simulink model "orbit_propogator_simulink"  (R2023b)
settings: Solver=FixedStepAuto  StartTime=0  StopTime=5929*3  FixedStep=50  RelTol=1e-3
settings Model: Creator=annahylbert  LastModifiedBy=annahylbert

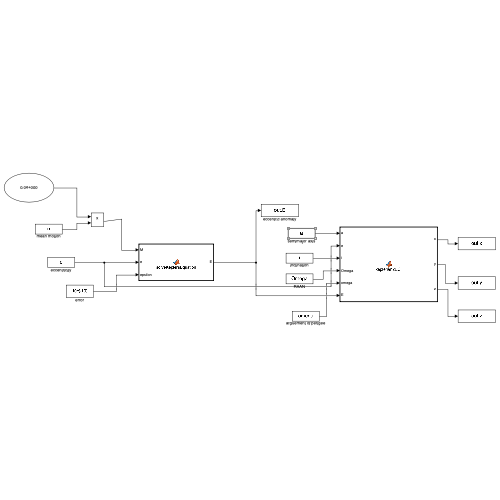
[thumbnail: Simulink's stored preview of the top-level diagram]
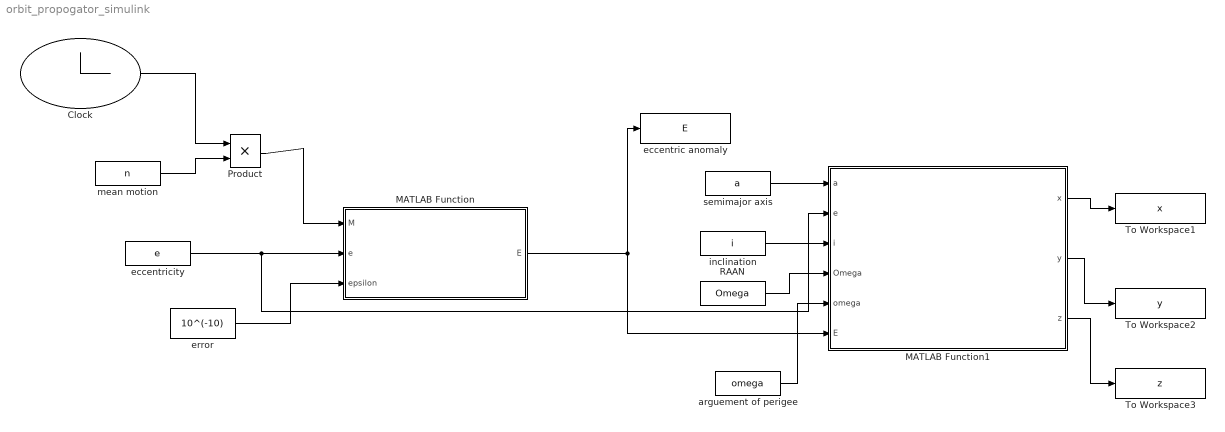
== system orbit_propogator_simulink ==
  Clock : Clock
      settings: Decimation=99999999
  MATLAB Function : MATLAB Function  TreatAsAtomicUnit=on
  MATLAB Function1 : MATLAB Function  TreatAsAtomicUnit=on
  Product : Product
  RAAN : FromWorkspace  VariableName=Omega
  To Workspace1 : ToWorkspace  VariableName=x  SaveFormat=Timeseries  SampleTime=-1
  To Workspace2 : ToWorkspace  VariableName=y  SaveFormat=Timeseries  SampleTime=-1
  To Workspace3 : ToWorkspace  VariableName=z  SaveFormat=Timeseries  SampleTime=-1
  arguement of perigee : FromWorkspace  VariableName=omega
  eccentric anomaly : ToWorkspace  VariableName=E  SaveFormat=Timeseries  SampleTime=-1
  eccentricity : FromWorkspace  VariableName=e
  error : Constant  Value=10^(-10)
  inclination : FromWorkspace  VariableName=i
  mean motion : FromWorkspace  VariableName=n
  semimajor axis : FromWorkspace  VariableName=a  OutDataTypeStr=double
  wires:
  eccentricity/1 -> MATLAB Function1/2(e), MATLAB Function/2(e)
  Product/1 -> MATLAB Function/1(M)
  mean motion/1 -> Product/2
  Clock/1 -> Product/1
  error/1 -> MATLAB Function/3(epsilon)
  MATLAB Function/1(E) -> MATLAB Function1/6(E), eccentric anomaly/1
  semimajor axis/1 -> MATLAB Function1/1(a)
  MATLAB Function1/1(x) -> To Workspace1/1
  MATLAB Function1/2(y) -> To Workspace2/1
  MATLAB Function1/3(z) -> To Workspace3/1
  inclination/1 -> MATLAB Function1/3(i)
  RAAN/1 -> MATLAB Function1/4(Omega)
  arguement of perigee/1 -> MATLAB Function1/5(omega)

== matlab function orbit_propogator_simulink/MATLAB Function1 ==
  data: a input; x output; e input; i input; Omega input; omega input; E input; y output; z output
function [x,y,z]  = keplerian2ECI(a, e, i, Omega, omega, E)
    % Constants
    mu = 3.986e5; % Earth's gravitational parameter (km^3/s^2)

    % Convert orbital elements from degrees to radians
    i = deg2rad(i);
    Omega = deg2rad(Omega);
    omega = deg2rad(omega);

    % Calculate position and velocity in the perifocal coordinate system
    n = sqrt(mu/a^3);
    r_perifocal = [a*(cos(E) - e); a*sin(E)*sqrt(1-e^2); 0];
    v_perifocal = a*n/(1-e*cos(E)) * [-sin(E); cos(E)*sqrt(1-e^2); 0];

    % Rotation matrices
    R3_Omega = [cos(-Omega) sin(-Omega) 0;
                -sin(-Omega) cos(-Omega) 0;
                0 0 1];
    R1_i = [1 0 0;
            0 cos(-i) sin(-i);
            0 -sin(-i) cos(-i)];
    R3_omega = [cos(-omega) sin(-omega) 0;
                -sin(-omega) cos(-omega) 0;
                0 0 1];

    % Transformation to ECI
    Q_perifocal2ECI = R3_Omega * R1_i * R3_omega;
    rECI = Q_perifocal2ECI * r_perifocal;
    x = rECI(1);
    y = rECI(2);
    z = rECI(3);
end

== matlab function orbit_propogator_simulink/MATLAB Function ==
  data: M input; E output; e input; epsilon input
function E = solveKeplersEquation(M, e, epsilon)
    E = M; % Initial Guess
    while true
        E_new = E - (E - e*sin(E) - M) / (1 - e*cos(E)); % Newton-Raphson iteration
        if abs(E_new - E) < epsilon
            break; % Convergence reached
        end
        E = E_new;
    end
end
